simulink model "DSM_example"  (R2018a)
settings: Solver=VariableStepAuto  StartTime=0.0  StopTime=10  RelTol=1e-3
settings Model: Creator=86188  LastModifiedBy=86188

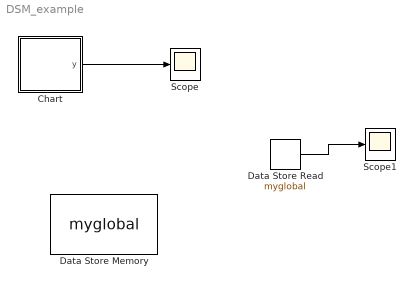
== system DSM_example ==
  Chart : Stateflow chart  TreatAsAtomicUnit=on
  Data Store Memory : DataStoreMemory  DataStoreName=myglobal  ReadBeforeWriteMsg=warning  WriteAfterWriteMsg=warning  WriteAfterReadMsg=warning  InitialValue=[0,0]  ShowAdditionalParam=off  OutDataTypeStr=double
  Data Store Read : DataStoreRead  DataStoreName=myglobal
  Scope : Scope
  Scope1 : Scope
  wires:
  Chart/1(y) -> Scope/1
  Data Store Read/1 -> Scope1/1

== stateflow chart DSM_example/Chart ==
  state A
    en: f("en_A");
    [myglobal(1)]=duA()
    du:f("du_A");
    myglobal(1) = myglobal(1) +1;
    y=myglobal(1) ;
  state B
    en:f("en_B");
    myglobal(2)=0;
    du:
    myglobal(2)= myglobal(2)-1;
    y=myglobal(2);
  (default) -> A
  A -> B : [u<0]
  B -> A : [u>=0]
  data: y1 function_output; s function_input; y output =0; myglobal data_store_memory; u local =2; x local
  function y1 =duA:
    | function y1 =duA
    | y1=3;
  function f(s):
    | function f(s)
    |   fprintf(s+"\n");
